simulink model "ModelForAdapt"  (R2020a)
settings: Solver=VariableStepAuto  StartTime=0.0  StopTime=10.0  RelTol=1e-3
InitFcn:
  | addpath('dynamics\')
  | parameters
undefined symbols (not defined in the file or in its folder): A, B, C, E, t_sample, x_0
settings Model: Creator=micha  LastModifiedBy=micha

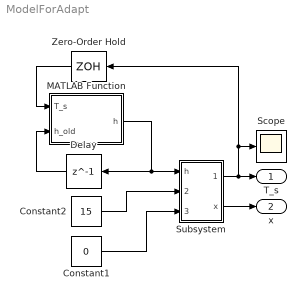
== system ModelForAdapt ==
  Constant1 : Constant  Value=0
  Constant2 : Constant  Value=15
  Delay : Delay  DelayLength=1  SampleTime=t_sample
  MATLAB Function : MATLAB Function  TreatAsAtomicUnit=on
  Scope : Scope
  Subsystem : Subsystem
  Zero-Order Hold : ZeroOrderHold  SampleTime=-1
  T_s : Outport
  x : Outport  Port=2
  wires:
  Subsystem/2(x) -> x/1
  Constant1/1 -> Subsystem/3(phi_s)
  Constant2/1 -> Subsystem/2(T_a)
  MATLAB Function/1(h) -> Delay/1, Subsystem/1(h)
  Subsystem/1(T_s) -> Zero-Order Hold/1, Scope/1, T_s/1
  Zero-Order Hold/1 -> MATLAB Function/1(T_s)
  Delay/1 -> MATLAB Function/2(h_old)

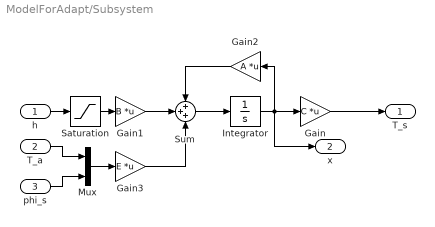
== system ModelForAdapt/Subsystem ==
  h : Inport
  T_a : Inport  Port=2
  phi_s : Inport  Port=3
  Gain : Gain  InitFcn=parameters  Gain=C  Multiplication=Matrix(K*u)
  Gain1 : Gain  Gain=B  Multiplication=Matrix(K*u)
  Gain2 : Gain  Gain=A  Multiplication=Matrix(K*u)
  Gain3 : Gain  Gain=E  Multiplication=Matrix(K*u)
  Integrator : Integrator  InitialCondition=x_0
  Mux : Mux  Inputs=2
  Saturation : Saturate  UpperLimit=1  LowerLimit=0
  Sum : Sum  Inputs=+++
  T_s : Outport
  x : Outport  Port=2
  wires:
  Saturation/1 -> Gain1/1
  Gain/1 -> T_s/1
  Integrator/1 -> x/1, Gain2/1, Gain/1
  Gain2/1 -> Sum/1
  T_a/1 -> Mux/1
  phi_s/1 -> Mux/2
  Mux/1 -> Gain3/1
  h/1 -> Saturation/1
  Gain3/1 -> Sum/3
  Sum/1 -> Integrator/1
  Gain1/1 -> Sum/2

== matlab function ModelForAdapt/MATLAB Function ==
  data: T_s input; h_old input; h output
function h = fcn(T_s, h_old)

if (T_s > 22 && h_old == 1)
    h = 0;
    return
elseif (T_s < 20 && h_old == 0)
    h = 1;
    return
end

h = h_old;
